simulink model "RPP_BankedDeePC"  (R2024a)
settings: Solver=FixedStepAuto  StartTime=0.0  StopTime=130  FixedStep=0.05  RelTol=1e-3
PostLoadFcn:
  | on_model_load
InitFcn:
  | on_model_start
StopFcn:
  | on_simulation_done
model workspace (MAT data in the model file):
  ActiveExperiment.Id = '1e727098-795b-40af-9168-30502f01196e'
  ActiveExperiment.Name = "Two steps"
  ActiveExperiment.Description = ""
  ActiveExperiment.ConstHorizonReference = 0
  ActiveExperiment.ComponentType = "scenario"
  ActiveExperiment.SimulationTime = 60
  ActiveExperiment.Subcomponents = "Disturbance"
  ActiveExperiment.Disturbance = struct()
  ActiveExperiment.SystemIc = [0; 0; 0; 0; 0; 0; 0; 0; 0; 0; 0; 0]
  ActiveExperiment.SystemParameterOverrides.payload_mass.timeseries__ = 1
  ActiveExperiment.SystemParameterOverrides.payload_mass.data = [0  0; 27  0]
  ActiveExperiment.Reference = '/home/luka/fer/csbenchlab_gym/envs/marine_otter_full/data/references/1e727098-795b-40af-9168-30502f01196e_ref.mat'
  ActiveExperiment.DisturbanceParameterOverrides = struct()
  ActiveExperiment.NumEvaluations = 1
  ActiveExperiment.RandomSeed = 42
  ActiveExperiment.SystemParams.payload_mass = timeseries
  ActiveExperiment.SystemParams.payload_mass.Name = 'unnamed'
  ActiveExperiment.SystemParams.payload_mass.DataInfo = tsdata.datametadata
  ActiveExperiment.SystemParams.payload_mass.DataInfo.Interpolation = tsdata.interpolation
  ActiveExperiment.SystemParams.payload_mass.DataInfo.Interpolation.Fhandle : function handle (value not decoded)
  ActiveExperiment.SystemParams.payload_mass.DataInfo.Interpolation.Name = 'linear'
  ActiveExperiment.SystemParams.payload_mass.TimeInfo = tsdata.timemetadata
  ActiveExperiment.SystemParams.payload_mass.TimeInfo.Length = 2
  ActiveExperiment.SystemParams.payload_mass.TimeInfo.DuplicateTimes = 0
  ActiveExperiment.SystemParams.payload_mass.TimeInfo.Time_ = [0; 27]
  ActiveExperiment.SystemParams.payload_mass.TimeInfo.Initialized = 1
  ActiveExperiment.SystemParams.payload_mass.QualityInfo = tsdata.qualmetadata
  ActiveExperiment.SystemParams.payload_mass.Data_ = [0; 0]
  ActiveExperiment.SystemParams.payload_location = timeseries
  ActiveExperiment.SystemParams.payload_location.Name = 'unnamed'
  ActiveExperiment.SystemParams.payload_location.DataInfo = tsdata.datametadata
  ActiveExperiment.SystemParams.payload_location.DataInfo.Interpolation = tsdata.interpolation
  ActiveExperiment.SystemParams.payload_location.DataInfo.Interpolation.Fhandle : function handle (value not decoded)
  ActiveExperiment.SystemParams.payload_location.DataInfo.Interpolation.Name = 'linear'
  ActiveExperiment.SystemParams.payload_location.TimeInfo = tsdata.timemetadata
  ActiveExperiment.SystemParams.payload_location.TimeInfo.Length = 1
  ActiveExperiment.SystemParams.payload_location.TimeInfo.DuplicateTimes = 0
  ActiveExperiment.SystemParams.payload_location.TimeInfo.Time_ = 0
  ActiveExperiment.SystemParams.payload_location.TimeInfo.Initialized = 1
  ActiveExperiment.SystemParams.payload_location.QualityInfo = tsdata.qualmetadata
  ActiveExperiment.SystemParams.payload_location.Data_ = [0; 0; 0]
  ActiveExperiment.SystemParams.current_speed = timeseries
  ActiveExperiment.SystemParams.current_speed.Name = 'unnamed'
  ActiveExperiment.SystemParams.current_speed.DataInfo = tsdata.datametadata
  ActiveExperiment.SystemParams.current_speed.DataInfo.Interpolation = tsdata.interpolation
  ActiveExperiment.SystemParams.current_speed.DataInfo.Interpolation.Fhandle : function handle (value not decoded)
  ActiveExperiment.SystemParams.current_speed.DataInfo.Interpolation.Name = 'linear'
  ActiveExperiment.SystemParams.current_speed.TimeInfo = tsdata.timemetadata
  ActiveExperiment.SystemParams.current_speed.TimeInfo.Length = 1
  ActiveExperiment.SystemParams.current_speed.TimeInfo.DuplicateTimes = 0
  ActiveExperiment.SystemParams.current_speed.TimeInfo.Time_ = 0
  ActiveExperiment.SystemParams.current_speed.TimeInfo.Initialized = 1
  ActiveExperiment.SystemParams.current_speed.QualityInfo = tsdata.qualmetadata
  ActiveExperiment.SystemParams.current_speed.Data_ = 0
  ActiveExperiment.SystemParams.current_direction = timeseries
  ActiveExperiment.SystemParams.current_direction.Name = 'unnamed'
  ActiveExperiment.SystemParams.current_direction.DataInfo = tsdata.datametadata
  ActiveExperiment.SystemParams.current_direction.DataInfo.Interpolation = tsdata.interpolation
  ActiveExperiment.SystemParams.current_direction.DataInfo.Interpolation.Fhandle : function handle (value not decoded)
  ActiveExperiment.SystemParams.current_direction.DataInfo.Interpolation.Name = 'linear'
  ActiveExperiment.SystemParams.current_direction.TimeInfo = tsdata.timemetadata
  ActiveExperiment.SystemParams.current_direction.TimeInfo.Length = 1
  ActiveExperiment.SystemParams.current_direction.TimeInfo.DuplicateTimes = 0
  ActiveExperiment.SystemParams.current_direction.TimeInfo.Time_ = 0
  ActiveExperiment.SystemParams.current_direction.TimeInfo.Initialized = 1
  ActiveExperiment.SystemParams.current_direction.QualityInfo = tsdata.qualmetadata
  ActiveExperiment.SystemParams.current_direction.Data_ = 0
  ActiveExperiment.SystemParams.out_gain = timeseries
  ActiveExperiment.SystemParams.out_gain.Name = 'unnamed'
  ActiveExperiment.SystemParams.out_gain.DataInfo = tsdata.datametadata
  ActiveExperiment.SystemParams.out_gain.DataInfo.Interpolation = tsdata.interpolation
  ActiveExperiment.SystemParams.out_gain.DataInfo.Interpolation.Fhandle : function handle (value not decoded)
  ActiveExperiment.SystemParams.out_gain.DataInfo.Interpolation.Name = 'linear'
  ActiveExperiment.SystemParams.out_gain.TimeInfo = tsdata.timemetadata
  ActiveExperiment.SystemParams.out_gain.TimeInfo.Length = 1
  ActiveExperiment.SystemParams.out_gain.TimeInfo.DuplicateTimes = 0
  ActiveExperiment.SystemParams.out_gain.TimeInfo.Time_ = 0
  ActiveExperiment.SystemParams.out_gain.TimeInfo.Initialized = 1
  ActiveExperiment.SystemParams.out_gain.QualityInfo = tsdata.qualmetadata
  ActiveExperiment.SystemParams.out_gain.Data_ = 1
  Experiments(1).Id = '1e1e735a-ca72-47f3-9e23-ef054322de06'
  Experiments(1).Name = "Five steps perturbed high noise"
  Experiments(1).Description = ""
  Experiments(1).ConstHorizonReference = 0
  Experiments(1).ComponentType = "scenario"
  Experiments(1).SimulationTime = 60
  Experiments(1).Subcomponents = "Disturbance"
  Experiments(1).Disturbance.Id = 'd00b25fa-299c-4dde-a026-233da86bc131'
  Experiments(1).Disturbance.Name = ''
  Experiments(1).Disturbance.Description = ''
  Experiments(1).Disturbance.LibVersionHash = ''
  Experiments(1).Disturbance.Lib = 'csbenchlab'
  Experiments(1).Disturbance.LibVersion = '0.0.1'
  Experiments(1).Disturbance.PluginType = 'dist'
  Experiments(1).Disturbance.PluginName = 'Gauss'
  Experiments(1).Disturbance.PluginImplementation = 'mat'
  Experiments(1).Disturbance.ParentComponentId = '1e1e735a-ca72-47f3-9e23-ef054322de06'
  Experiments(1).Disturbance.ParentComponentName = 'Five steps perturbed high noise'
  Experiments(1).Disturbance.ParentComponentType = 'scenario'
  Experiments(1).Disturbance.ComponentType = 'disturbance'
  Experiments(1).Disturbance.DestinationPath = 'disturbances'
  Experiments(1).SystemIc = [0; 0; 0; 0; 0; 0; 0; 0; 0; 0; 0; 0]
  Experiments(1).SystemParameterOverrides.payload_mass.timeseries__ = 1
  Experiments(1).SystemParameterOverrides.payload_mass.data = [0  35; 27  35]
  Experiments(1).Reference = '/home/luka/fer/csbenchlab_gym/envs/marine_otter_full/data/references/1e1e735a-ca72-47f3-9e23-ef054322de06_ref.mat'
  Experiments(1).DisturbanceParameterOverrides = struct()
  Experiments(1).NumEvaluations = 1000
  Experiments(1).RandomSeed = 42
  Experiments(2).Id = '1e727098-795b-40af-9168-30502f01196e'
  Experiments(2).Name = "Two steps"
  Experiments(2).Description = ""
  Experiments(2).ConstHorizonReference = 0
  Experiments(2).ComponentType = "scenario"
  Experiments(2).SimulationTime = 60
  Experiments(2).Subcomponents = "Disturbance"
  Experiments(2).Disturbance = struct()
  Experiments(2).SystemIc = [0; 0; 0; 0; 0; 0; 0; 0; 0; 0; 0; 0]
  Experiments(2).SystemParameterOverrides.payload_mass.timeseries__ = 1
  Experiments(2).SystemParameterOverrides.payload_mass.data = [0  0; 27  0]
  Experiments(2).Reference = '/home/luka/fer/csbenchlab_gym/envs/marine_otter_full/data/references/1e727098-795b-40af-9168-30502f01196e_ref.mat'
  Experiments(2).DisturbanceParameterOverrides = struct()
  Experiments(2).NumEvaluations = 1
  Experiments(2).RandomSeed = 42
  Experiments(3).Id = '832a0fb6-0823-4b09-93b7-a1f8c841e784'
  Experiments(3).Name = "Sinuses"
  Experiments(3).Description = ""
  Experiments(3).ConstHorizonReference = 0
  Experiments(3).ComponentType = "scenario"
  Experiments(3).SimulationTime = 60
  Experiments(3).Subcomponents = "Disturbance"
  Experiments(3).Disturbance.Id = '6582568e-6a07-4ca1-973d-ce726013b9e5'
  Experiments(3).Disturbance.Name = ''
  Experiments(3).Disturbance.Description = ''
  Experiments(3).Disturbance.LibVersionHash = ''
  Experiments(3).Disturbance.Lib = 'csbenchlab'
  Experiments(3).Disturbance.LibVersion = '0.0.1'
  Experiments(3).Disturbance.PluginType = 'dist'
  Experiments(3).Disturbance.PluginName = 'Gauss'
  Experiments(3).Disturbance.PluginImplementation = 'mat'
  Experiments(3).Disturbance.ParentComponentId = '832a0fb6-0823-4b09-93b7-a1f8c841e784'
  Experiments(3).Disturbance.ParentComponentName = 'Sinuses'
  Experiments(3).Disturbance.ParentComponentType = 'scenario'
  Experiments(3).Disturbance.ComponentType = 'disturbance'
  Experiments(3).Disturbance.DestinationPath = 'disturbances'
  Experiments(3).SystemIc = [0; 0; 0; 0; 0; 0; 0; 0; 0; 0; 0; 0]
  Experiments(3).SystemParameterOverrides.payload_mass.timeseries__ = 1
  Experiments(3).SystemParameterOverrides.payload_mass.data = [0  35; 12  35]
  Experiments(3).Reference = '/home/luka/fer/csbenchlab_gym/envs/marine_otter_full/data/references/832a0fb6-0823-4b09-93b7-a1f8c841e784_ref.mat'
  Experiments(3).DisturbanceParameterOverrides = struct()
  Experiments(3).NumEvaluations = 1000
  Experiments(3).RandomSeed = 42
  Experiments(4).Id = '85ae8ae8-3421-447e-86e6-f1860a57dbe5'
  Experiments(4).Name = "Two steps high noise"
  Experiments(4).Description = ""
  Experiments(4).ConstHorizonReference = 0
  Experiments(4).ComponentType = "scenario"
  Experiments(4).SimulationTime = 60
  Experiments(4).Subcomponents = "Disturbance"
  Experiments(4).Disturbance.Id = 'ccaeaedb-34fb-4469-93e3-0e771cb356d7'
  Experiments(4).Disturbance.Name = 'New Disturbance'
  Experiments(4).Disturbance.Description = ''
  Experiments(4).Disturbance.LibVersionHash = ''
  Experiments(4).Disturbance.Lib = 'csbenchlab'
  Experiments(4).Disturbance.LibVersion = '0.0.1'
  Experiments(4).Disturbance.PluginType = 'dist'
  Experiments(4).Disturbance.PluginName = 'Gauss'
  Experiments(4).Disturbance.PluginImplementation = 'mat'
  Experiments(4).Disturbance.ParentComponentId = '85ae8ae8-3421-447e-86e6-f1860a57dbe5'
  Experiments(4).Disturbance.ParentComponentType = 'scenario'
  Experiments(4).Disturbance.ComponentType = 'disturbance'
  Experiments(4).Disturbance.ParentComponentName = 'Two steps high noise'
  Experiments(4).SystemIc = [0; 0; 0; 0; 0; 0; 0; 0; 0; 0; 0; 0]
  Experiments(4).SystemParameterOverrides.payload_mass.timeseries__ = 1
  Experiments(4).SystemParameterOverrides.payload_mass.data = [0  0; 30  20]
  Experiments(4).SystemParameterOverrides.payload_location.timeseries__ = 1
  Experiments(4).SystemParameterOverrides.payload_location.data = [0 0 -0.15 0]
  Experiments(4).SystemParameterOverrides.current_speed = 0.2
  Experiments(4).SystemParameterOverrides.current_direction = 0.1
  Experiments(4).Reference = '/home/luka/fer/csbenchlab_gym/envs/marine_otter_full/data/references/85ae8ae8-3421-447e-86e6-f1860a57dbe5_ref.mat'
  Experiments(4).DisturbanceParameterOverrides = struct()
  Experiments(4).NumEvaluations = 1
  Experiments(4).RandomSeed = 42
  Experiments(5).Id = '9caafca7-6b3d-4fd5-b43b-2d0badebda60'
  Experiments(5).Name = "Five steps perturbed"
  Experiments(5).Description = ""
  Experiments(5).ConstHorizonReference = 0
  Experiments(5).ComponentType = "scenario"
  Experiments(5).SimulationTime = 60
  Experiments(5).Subcomponents = "Disturbance"
  Experiments(5).Disturbance.Id = '941af73e-12e7-42cf-853d-f79bb40068e7'
  Experiments(5).Disturbance.Name = ''
  Experiments(5).Disturbance.Description = ''
  Experiments(5).Disturbance.LibVersionHash = ''
  Experiments(5).Disturbance.Lib = 'csbenchlab'
  Experiments(5).Disturbance.LibVersion = '0.0.1'
  Experiments(5).Disturbance.PluginType = 'dist'
  Experiments(5).Disturbance.PluginName = 'Gauss'
  Experiments(5).Disturbance.PluginImplementation = 'mat'
  Experiments(5).Disturbance.ParentComponentId = '9caafca7-6b3d-4fd5-b43b-2d0badebda60'
  Experiments(5).Disturbance.ParentComponentName = 'Five steps perturbed'
  Experiments(5).Disturbance.ParentComponentType = 'scenario'
  Experiments(5).Disturbance.ComponentType = 'disturbance'
  Experiments(5).Disturbance.DestinationPath = 'disturbances'
  Experiments(5).SystemIc = [0; 0; 0; 0; 0; 0; 0; 0; 0; 0; 0; 0]
  Experiments(5).SystemParameterOverrides.payload_mass.timeseries__ = 1
  Experiments(5).SystemParameterOverrides.payload_mass.data = [0  0; 27  0]
  Experiments(5).Reference = '/home/luka/fer/csbenchlab_gym/envs/marine_otter_full/data/references/9caafca7-6b3d-4fd5-b43b-2d0badebda60_ref.mat'
  Experiments(5).DisturbanceParameterOverrides = struct()
  Experiments(5).NumEvaluations = 1000
  Experiments(5).RandomSeed = 42
  Experiments(6).Id = 'd997722b-b22e-4a88-a68f-d421073cfd81'
  Experiments(6).Name = "Sinuses high noise"
  Experiments(6).Description = ""
  Experiments(6).ConstHorizonReference = 0
  Experiments(6).ComponentType = "scenario"
  Experiments(6).SimulationTime = 60
  Experiments(6).Subcomponents = "Disturbance"
  Experiments(6).Disturbance.Id = 'e3fab669-38a8-480e-9185-300544970487'
  Experiments(6).Disturbance.Name = ''
  Experiments(6).Disturbance.Description = ''
  Experiments(6).Disturbance.LibVersionHash = ''
  Experiments(6).Disturbance.Lib = 'csbenchlab'
  Experiments(6).Disturbance.LibVersion = '0.0.1'
  Experiments(6).Disturbance.PluginType = 'dist'
  Experiments(6).Disturbance.PluginName = 'Gauss'
  Experiments(6).Disturbance.PluginImplementation = 'mat'
  Experiments(6).Disturbance.ParentComponentId = 'd997722b-b22e-4a88-a68f-d421073cfd81'
  Experiments(6).Disturbance.ParentComponentName = 'Sinuses high noise'
  Experiments(6).Disturbance.ParentComponentType = 'scenario'
  Experiments(6).Disturbance.ComponentType = 'disturbance'
  Experiments(6).Disturbance.DestinationPath = 'disturbances'
  Experiments(6).SystemIc = [0; 0; 0; 0; 0; 0; 0; 0; 0; 0; 0; 0]
  Experiments(6).SystemParameterOverrides.payload_mass.timeseries__ = 1
  Experiments(6).SystemParameterOverrides.payload_mass.data = [0  35; 12  35]
  Experiments(6).Reference = '/home/luka/fer/csbenchlab_gym/envs/marine_otter_full/data/references/d997722b-b22e-4a88-a68f-d421073cfd81_ref.mat'
  Experiments(6).DisturbanceParameterOverrides = struct()
  Experiments(6).NumEvaluations = 1000
  Experiments(6).RandomSeed = 42
  GlobalReference = 0
  RPP_BankedDeePC_CS_Controller_BankedDeePC_d_data.Ts = 0.05
  RPP_BankedDeePC_CS_Controller_BankedDeePC_d_data.T = 100
  RPP_BankedDeePC_CS_Controller_BankedDeePC_d_data.m = 2
  RPP_BankedDeePC_CS_Controller_BankedDeePC_d_data.p = 2
  RPP_BankedDeePC_CS_Controller_BankedDeePC_d_data.L = 12
  RPP_BankedDeePC_CS_Controller_BankedDeePC_d_data.Tini = 5
  RPP_BankedDeePC_CS_Controller_BankedDeePC_d_data.vel_stop_idx = 2
  RPP_BankedDeePC_CS_Controller_BankedDeePC_d_data.idx.m = 2
  RPP_BankedDeePC_CS_Controller_BankedDeePC_d_data.idx.p = 2
  RPP_BankedDeePC_CS_Controller_BankedDeePC_d_data.idx.L = 12
  RPP_BankedDeePC_CS_Controller_BankedDeePC_d_data.idx.Tini = 5
  RPP_BankedDeePC_CS_Controller_BankedDeePC_d_data.idx.uini_v.b = 1
  RPP_BankedDeePC_CS_Controller_BankedDeePC_d_data.idx.uini_v.e = 10
  RPP_BankedDeePC_CS_Controller_BankedDeePC_d_data.idx.uini_v.sz = 10
  RPP_BankedDeePC_CS_Controller_BankedDeePC_d_data.idx.uini_v.r = [1 2 3 4 5 6 7 8 9 10]
  RPP_BankedDeePC_CS_Controller_BankedDeePC_d_data.idx.u_v.b = 11
  RPP_BankedDeePC_CS_Controller_BankedDeePC_d_data.idx.u_v.e = 34
  RPP_BankedDeePC_CS_Controller_BankedDeePC_d_data.idx.u_v.sz = 24
  RPP_BankedDeePC_CS_Controller_BankedDeePC_d_data.idx.u_v.r = [11 12 13 14 15 16 17 18 19 20 21 22 23 24 25 26 27 28 29 30 31 32 33 34]
  RPP_BankedDeePC_CS_Controller_BankedDeePC_d_data.idx.yini_v.b = 35
  RPP_BankedDeePC_CS_Controller_BankedDeePC_d_data.idx.yini_v.e = 44
  RPP_BankedDeePC_CS_Controller_BankedDeePC_d_data.idx.yini_v.sz = 10
  RPP_BankedDeePC_CS_Controller_BankedDeePC_d_data.idx.yini_v.r = [35 36 37 38 39 40 41 42 43 44]
  RPP_BankedDeePC_CS_Controller_BankedDeePC_d_data.idx.y_v.b = 45
  RPP_BankedDeePC_CS_Controller_BankedDeePC_d_data.idx.y_v.e = 68
  RPP_BankedDeePC_CS_Controller_BankedDeePC_d_data.idx.y_v.sz = 24
  RPP_BankedDeePC_CS_Controller_BankedDeePC_d_data.idx.y_v.r = [45 46 47 48 49 50 51 52 53 54 55 56 57 58 59 60 61 62 63 64 65 66 67 68]
  RPP_BankedDeePC_CS_Controller_BankedDeePC_d_data.idx.u.b = 1
  RPP_BankedDeePC_CS_Controller_BankedDeePC_d_data.idx.u.e = 24
  RPP_BankedDeePC_CS_Controller_BankedDeePC_d_data.idx.u.sz = 24
  RPP_BankedDeePC_CS_Controller_BankedDeePC_d_data.idx.u.r = [1 2 3 4 5 6 7 8 9 10 11 12 13 14 15 16 17 18 19 20 21 22 23 24]
  RPP_BankedDeePC_CS_Controller_BankedDeePC_d_data.idx.y.b = 25
  RPP_BankedDeePC_CS_Controller_BankedDeePC_d_data.idx.y.e = 48
  RPP_BankedDeePC_CS_Controller_BankedDeePC_d_data.idx.y.sz = 24
  RPP_BankedDeePC_CS_Controller_BankedDeePC_d_data.idx.y.r = [25 26 27 28 29 30 31 32 33 34 35 36 37 38 39 40 41 42 43 44 45 46 47 48]
  RPP_BankedDeePC_CS_Controller_BankedDeePC_d_data.idx.s.b = 49
  RPP_BankedDeePC_CS_Controller_BankedDeePC_d_data.idx.s.e = 82
  RPP_BankedDeePC_CS_Controller_BankedDeePC_d_data.idx.s.sz = 34
  RPP_BankedDeePC_CS_Controller_BankedDeePC_d_data.idx.s.r = [49 50 51 52 53 54 55 56 57 58 59 60 61 62 63 64 65 66 67 68 69 70 71 72 73 74 75 76 77 78 79 80 81 82]
  RPP_BankedDeePC_CS_Controller_BankedDeePC_d_data.idx.A_v.b = 1
  RPP_BankedDeePC_CS_Controller_BankedDeePC_d_data.idx.A_v.e = 68
  RPP_BankedDeePC_CS_Controller_BankedDeePC_d_data.idx.A_v.sz = 68
  RPP_BankedDeePC_CS_Controller_BankedDeePC_d_data.idx.A_v.r = [1 2 3 4 5 6 7 8 9 10 11 12 13 14 15 16 17 18 19 20 21 22 23 24 25 26 27 28 29 30 31 32 33 34 35 36 37 38 39 40 41 42 43 44 45 46 47 48 49 50 51 52 53 54 55 56 57 58 59 60 61 62 63 64 65 66 67 68]
  RPP_BankedDeePC_CS_Controller_BankedDeePC_d_data.idx.yterm.b = 83
  RPP_BankedDeePC_CS_Controller_BankedDeePC_d_data.idx.yterm.e = 84
  RPP_BankedDeePC_CS_Controller_BankedDeePC_d_data.idx.yterm.sz = 2
  RPP_BankedDeePC_CS_Controller_BankedDeePC_d_data.idx.yterm.r = [83 84]
  RPP_BankedDeePC_CS_Controller_BankedDeePC_d_data.idx.uterm.b = 85
  RPP_BankedDeePC_CS_Controller_BankedDeePC_d_data.idx.uterm.e = 86
  RPP_BankedDeePC_CS_Controller_BankedDeePC_d_data.idx.uterm.sz = 2
  RPP_BankedDeePC_CS_Controller_BankedDeePC_d_data.idx.uterm.r = [85 86]
  RPP_BankedDeePC_CS_Controller_BankedDeePC_d_data.idx.uterm_v.b = 72
  RPP_BankedDeePC_CS_Controller_BankedDeePC_d_data.idx.uterm_v.e = 73
  RPP_BankedDeePC_CS_Controller_BankedDeePC_d_data.idx.uterm_v.sz = 2
  RPP_BankedDeePC_CS_Controller_BankedDeePC_d_data.idx.uterm_v.r = [72 73]
  RPP_BankedDeePC_CS_Controller_BankedDeePC_d_data.idx.yterm_v.b = 70
  RPP_BankedDeePC_CS_Controller_BankedDeePC_d_data.idx.yterm_v.e = 71
  RPP_BankedDeePC_CS_Controller_BankedDeePC_d_data.idx.yterm_v.sz = 2
  RPP_BankedDeePC_CS_Controller_BankedDeePC_d_data.idx.yterm_v.r = [70 71]
  RPP_BankedDeePC_CS_Controller_BankedDeePC_d_data.idx.affine_v.b = 69
  RPP_BankedDeePC_CS_Controller_BankedDeePC_d_data.idx.affine_v.e = 69
  RPP_BankedDeePC_CS_Controller_BankedDeePC_d_data.idx.affine_v.sz = 1
  RPP_BankedDeePC_CS_Controller_BankedDeePC_d_data.idx.affine_v.r = 69
  RPP_BankedDeePC_CS_Controller_BankedDeePC_d_data.idx.total_constraints = 5
  RPP_BankedDeePC_CS_Controller_BankedDeePC_d_data.idx.term_v.b = 69
  RPP_BankedDeePC_CS_Controller_BankedDeePC_d_data.idx.term_v.e = 73
  RPP_BankedDeePC_CS_Controller_BankedDeePC_d_data.idx.term_v.sz = 5
  RPP_BankedDeePC_CS_Controller_BankedDeePC_d_data.idx.term_v.r = [69 70 71 72 73]
  RPP_BankedDeePC_CS_Controller_BankedDeePC_d_data.idx.a.b = 87
  RPP_BankedDeePC_CS_Controller_BankedDeePC_d_data.idx.a.e = 170
  RPP_BankedDeePC_CS_Controller_BankedDeePC_d_data.idx.a.sz = 84
  RPP_BankedDeePC_CS_Controller_BankedDeePC_d_data.idx.a.r = [87 88 89 90 91 92 93 94 95 96 97 98 99 100 101 102 103 104 105 106 107 108 109 110 111 112 113 114 115 116 117 118 119 120 121 122 123 124 125 126 127 128 129 130 131 132 133 134 135 136 137 138 139 140 141 142 143 144 145 146 147 148 149 150 151 152 153 154 155 156 157 158 159 160 161 162 163 164 165 166 167 168 169 170]
  RPP_BankedDeePC_CS_Controller_BankedDeePC_d_data.idx.state.b = 1
  RPP_BankedDeePC_CS_Controller_BankedDeePC_d_data.idx.state.e = 170
  RPP_BankedDeePC_CS_Controller_BankedDeePC_d_data.idx.state.sz = 170
  RPP_BankedDeePC_CS_Controller_BankedDeePC_d_data.idx.state.r = [1 2 3 4 5 6 7 8 9 10 11 12 13 14 15 16 17 18 19 20 21 22 23 24 25 26 27 28 29 30 31 32 33 34 35 36 37 38 39 40 41 42 43 44 45 46 47 48 49 50 51 52 53 54 55 56 57 58 59 60 61 62 63 64 65 66 67 68 69 70 71 72 73 74 75 76 77 78 79 80 81 82 83 84 85 86 87 88 89 90 91 92 93 94 95 96 97 98 99 100 101 102 103 104 105 106 107 108 109 110 111 112 113 114 115 116 117 118 119 120 121 122 123 124 125 126 127 128 129 130 131 132 133 134 135 136 137 138 139 140 141 142 143 144 145 146 147 148 149 150 151 152 153 154 155 156 157 158 159 160 161 162 163 164 165 166 167 168 169 170]
  RPP_BankedDeePC_CS_Controller_BankedDeePC_d_data.idx.u_lt.b = 1
  RPP_BankedDeePC_CS_Controller_BankedDeePC_d_data.idx.u_lt.e = 48
  RPP_BankedDeePC_CS_Controller_BankedDeePC_d_data.idx.u_lt.sz = 48
  RPP_BankedDeePC_CS_Controller_BankedDeePC_d_data.idx.u_lt.r = [1 2 3 4 5 6 7 8 9 10 11 12 13 14 15 16 17 18 19 20 21 22 23 24 25 26 27 28 29 30 31 32 33 34 35 36 37 38 39 40 41 42 43 44 45 46 47 48]
  RPP_BankedDeePC_CS_Controller_BankedDeePC_d_data.idx.y_lt.b = -1
  RPP_BankedDeePC_CS_Controller_BankedDeePC_d_data.idx.y_lt.e = -1
  RPP_BankedDeePC_CS_Controller_BankedDeePC_d_data.idx.y_lt.sz = 1
  RPP_BankedDeePC_CS_Controller_BankedDeePC_d_data.idx.y_lt.r = -1
  RPP_BankedDeePC_CS_Controller_BankedDeePC_d_data.x_op_u = [0; 0; 0; 0; 0; 0; 0; 0; 0; 0; 0; 0; 0; 0; 0; 0; 0; 0; 0; 0; 0; 0; 0; 0]
  RPP_BankedDeePC_CS_Controller_BankedDeePC_d_data.x_op_y = [0; 0; 0; 0; 0; 0; 0; 0; 0; 0; 0; 0; 0; 0; 0; 0; 0; 0; 0; 0; 0; 0; 0; 0]
  RPP_BankedDeePC_CS_Controller_BankedDeePC_d_data.x_op_g = [0; 0; 0; 0; 0; 0; 0; 0; 0; 0; 0; 0; 0; 0; 0; 0; 0; 0; 0; 0; 0; 0; 0; 0; 0; 0; 0; 0; 0; 0; 0; 0; 0; 0; 0; 0; 0; 0; 0; 0; 0; 0; 0; 0; 0; 0; 0; 0; 0; 0; 0; 0; 0; 0; 0; 0; 0; 0; 0; 0; 0; 0; 0; 0; 0; 0; 0; 0; 0; 0; 0; 0; 0; 0; 0; 0; 0; 0; 0; 0; 0; 0; 0; 0]
  RPP_BankedDeePC_CS_Controller_BankedDeePC_d_data.uini = [0; 0; 0; 0; 0; 0; 0; 0; 0; 0]
  RPP_BankedDeePC_CS_Controller_BankedDeePC_d_data.yini = [0; 0; 0; 0; 0; 0; 0; 0; 0; 0]
  RPP_BankedDeePC_CS_Controller_BankedDeePC_d_data.A = [0 0 0 0 0 0 0 0 0 0 -1 0 ... (12410 elements, 73x170)]
  RPP_BankedDeePC_CS_Controller_BankedDeePC_d_data.b = [0; 0; 0; 0; 0; 0; 0; 0; 0; 0; 0; 0; 0; 0; 0; 0; 0; 0; 0; 0; 0; 0; 0; 0; 0; 0; 0; 0; 0; 0; 0; 0; 0; 0; 0; 0; 0; 0; 0; 0; 0; 0; 0; 0; 0; 0; 0; 0; 0; 0; 0; 0; 0; 0; 0; 0; 0; 0; 0; 0; 0; 0; 0; 0; 0; 0; 0; 0; 1; 0; 0; 0; 0]
  RPP_BankedDeePC_CS_Controller_BankedDeePC_d_data.A_lt = [1 0 -1 0 -1 0 1 0 0 0 0 0 ... (8160 elements, 48x170)]
  RPP_BankedDeePC_CS_Controller_BankedDeePC_d_data.b_lt = [0.2; 0.2; 0.2; 0.2; 0.2; 0.2; 0.2; 0.2; 0.2; 0.2; 0.2; 0.2; 0.2; 0.2; 0.2; 0.2; 0.2; 0.2; 0.2; 0.2; 0.2; 0.2; 0.2; 0.2; 0.2; 0.2; 0.2; 0.2; 0.2; 0.2; 0.2; 0.2; 0.2; 0.2; 0.2; 0.2; 0.2; 0.2; 0.2; 0.2; 0.2; 0.2; 0.2; 0.2; 0.2; 0.2; 0.2; 0.2]
  RPP_BankedDeePC_CS_Controller_BankedDeePC_d_data.optim_T = [0.0666666666667 0 0 0 0 0 0 0 0 0 0 0 ... (28900 elements, 170x170)]
  RPP_BankedDeePC_CS_Controller_BankedDeePC_d_data.optim_f = [0; 0; 0; 0; 0; 0; 0; 0; 0; 0; 0; 0; 0; 0; 0; 0; 0; 0; 0; 0; 0; 0; 0; 0; 0; 0; 0; 0; 0; 0; 0; 0; 0; 0; 0; 0; 0; 0; 0; 0; 0; 0; 0; 0; 0; 0; 0; 0; 0; 0; 0; 0; 0; 0; 0; 0; 0; 0; 0; 0; 0; 0; 0; 0; 0; 0; 0; 0; 0; 0; 0; 0; 0; 0; 0; 0; 0; 0; 0; 0; 0; 0; 0; 0; 0; 0; 0; 0; 0; 0; 0; 0; 0; 0; 0; 0; 0; 0; 0; 0; 0; 0; 0; 0; 0; 0; 0; 0; 0; 0; 0; 0; 0; 0; 0; 0; 0; 0; 0; 0; 0; 0; 0; 0; 0; 0; 0; 0; 0; 0; 0; 0; 0; 0; 0; 0; 0; 0; 0; 0; 0; 0; 0; 0; 0; 0; 0; 0; 0; 0; 0; 0; 0; 0; 0; 0; 0; 0; 0; 0; 0; 0; 0; 0; 0; 0; 0; 0; 0; 0]
  RPP_BankedDeePC_CS_Controller_BankedDeePC_d_data.x_op = [0; 0; 0; 0; 0; 0; 0; 0; 0; 0; 0; 0; 0; 0; 0; 0; 0; 0; 0; 0; 0; 0; 0; 0; 0; 0; 0; 0; 0; 0; 0; 0; 0; 0; 0; 0; 0; 0; 0; 0; 0; 0; 0; 0; 0; 0; 0; 0; 0; 0; 0; 0; 0; 0; 0; 0; 0; 0; 0; 0; 0; 0; 0; 0; 0; 0; 0; 0; 0; 0; 0; 0; 0; 0; 0; 0; 0; 0; 0; 0; 0; 0; 0; 0; 0; 0; 0; 0; 0; 0; 0; 0; 0; 0; 0; 0; 0; 0; 0; 0; 0; 0; 0; 0; 0; 0; 0; 0; 0; 0; 0; 0; 0; 0; 0; 0; 0; 0; 0; 0; 0; 0; 0; 0; 0; 0; 0; 0; 0; 0; 0; 0; 0; 0; 0; 0; 0; 0; 0; 0; 0; 0; 0; 0; 0; 0; 0; 0; 0; 0; 0; 0; 0; 0; 0; 0; 0; 0; 0; 0; 0; 0; 0; 0; 0; 0; 0; 0; 0; 0]
  RPP_BankedDeePC_CS_Controller_BankedDeePC_d_data.lb = [-Inf; -Inf; -Inf; -Inf; -Inf; -Inf; -Inf; -Inf; -Inf; -Inf; -Inf; -Inf; -Inf; -Inf; -Inf; -Inf; -Inf; -Inf; -Inf; -Inf; -Inf; -Inf; -Inf; -Inf; -Inf; -Inf; -Inf; -Inf; -Inf; -Inf; -Inf; -Inf; -Inf; -Inf; -Inf; -Inf; -Inf; -Inf; -Inf; -Inf; -Inf; -Inf; -Inf; -Inf; -Inf; -Inf; -Inf; -Inf; -Inf; -Inf; -Inf; -Inf; -Inf; -Inf; -Inf; -Inf; -Inf; -Inf; -Inf; -Inf; -Inf; -Inf; -Inf; -Inf; -Inf; -Inf; -Inf; -Inf; -Inf; -Inf; -Inf; -Inf; -Inf; -Inf; -Inf; -Inf; -Inf; -Inf; -Inf; -Inf; -Inf; -Inf; -Inf; -Inf; -Inf; -Inf; -Inf; -Inf; -Inf; -Inf; -Inf; -Inf; -Inf; -Inf; -Inf; -Inf; -Inf; -Inf; -Inf; -Inf; -Inf; -Inf; -Inf; -Inf; -Inf; -Inf; -Inf; -Inf; -Inf; -Inf; -Inf; -Inf; -Inf; -Inf; -Inf; -Inf; -Inf; -Inf; -Inf; -Inf; -Inf; -Inf; -Inf; -Inf; -Inf; -Inf; -Inf; -Inf; -Inf; -Inf; -Inf; -Inf; -Inf; -Inf; -Inf; -Inf; -Inf; -Inf; -Inf; -Inf; -Inf; -Inf; -Inf; -Inf; -Inf; -Inf; -Inf; -Inf; -Inf; -Inf; -Inf; -Inf; -Inf; -Inf; -Inf; -Inf; -Inf; -Inf; -Inf; -Inf; -Inf; -Inf; -Inf; -Inf; -Inf; -Inf; -Inf; -Inf; -Inf; -Inf]
  RPP_BankedDeePC_CS_Controller_BankedDeePC_d_data.ub = [Inf; Inf; Inf; Inf; Inf; Inf; Inf; Inf; Inf; Inf; Inf; Inf; Inf; Inf; Inf; Inf; Inf; Inf; Inf; Inf; Inf; Inf; Inf; Inf; Inf; Inf; Inf; Inf; Inf; Inf; Inf; Inf; Inf; Inf; Inf; Inf; Inf; Inf; Inf; Inf; Inf; Inf; Inf; Inf; Inf; Inf; Inf; Inf; Inf; Inf; Inf; Inf; Inf; Inf; Inf; Inf; Inf; Inf; Inf; Inf; Inf; Inf; Inf; Inf; Inf; Inf; Inf; Inf; Inf; Inf; Inf; Inf; Inf; Inf; Inf; Inf; Inf; Inf; Inf; Inf; Inf; Inf; Inf; Inf; Inf; Inf; Inf; Inf; Inf; Inf; Inf; Inf; Inf; Inf; Inf; Inf; Inf; Inf; Inf; Inf; Inf; Inf; Inf; Inf; Inf; Inf; Inf; Inf; Inf; Inf; Inf; Inf; Inf; Inf; Inf; Inf; Inf; Inf; Inf; Inf; Inf; Inf; Inf; Inf; Inf; Inf; Inf; Inf; Inf; Inf; Inf; Inf; Inf; Inf; Inf; Inf; Inf; Inf; Inf; Inf; Inf; Inf; Inf; Inf; Inf; Inf; Inf; Inf; Inf; Inf; Inf; Inf; Inf; Inf; Inf; Inf; Inf; Inf; Inf; Inf; Inf; Inf; Inf; Inf; Inf; Inf; Inf; Inf; Inf; Inf]
  RPP_BankedDeePC_CS_Controller_BankedDeePC_d_data.fval = 0
  RPP_BankedDeePC_CS_Controller_BankedDeePC_d_data.old_y_ref = [0; 0]
  RPP_BankedDeePC_CS_Controller_BankedDeePC_d_data.eta = [0; 0]
  RPP_BankedDeePC_CS_Controller_BankedDeePC_d_data.has_lt = 1
  callbacks = dictionary
  callbacks.data.Version = 1
  callbacks.data.IsKeyCombined = 1
  callbacks.data.IsValueCombined = 1
  callbacks.data.Key = ["on_start:31b52d05-ccc9-4eab-bb0e-3c80b4e6f477"; "on_start:f41ef9e4-ba34-416c-84b6-7794956a3c04"; "on_start:9c40ba40-a30c-4d47-b6ea-332d53085db4"; "on_start:a6a9c6d3-ff58-4f5d-b7b7-6a5809d04cef"; "on_start:59d3b695-31bd-4d38-a8d0-9c2b61ca3ebd"; "on_start:68187f7d-81f5-4756-96be-de0d65363a63"; "on_start:17c1b7c7-d1b2-4e6c-bab6-21ffb9ee4dcb"; "on_start:a5c8738f-8d38-4797-a21a-203fc6d46076"; "on_load:4a0d1010-4549-4d51-b3a5-602e7c932b45"; "on_start:4a0d1010-4549-4d51-b3a5-602e7c932b45"; "on_end:4a0d1010-4549-4d51-b3a5-602e7c932b45"]
  callbacks.data.Value{1}.external_function__ = 1
  callbacks.data.Value{1}.function = 'configure_controller_params'
  callbacks.data.Value{1}.backend = 'm'
  callbacks.data.Value{1}.kwargs = struct()
  callbacks.data.Value{2}.external_function__ = 1
  callbacks.data.Value{2}.function = 'configure_controller_params'
  callbacks.data.Value{2}.backend = 'm'
  callbacks.data.Value{2}.kwargs = struct()
  callbacks.data.Value{3}.external_function__ = 1
  callbacks.data.Value{3}.function = 'configure_controller_params'
  callbacks.data.Value{3}.backend = 'm'
  callbacks.data.Value{3}.kwargs = struct()
  callbacks.data.Value{4}.external_function__ = 1
  callbacks.data.Value{4}.function = 'configure_controller_params'
  callbacks.data.Value{4}.backend = 'm'
  callbacks.data.Value{4}.kwargs = struct()
  callbacks.data.Value{5}.external_function__ = 1
  callbacks.data.Value{5}.function = 'configure_controller_params'
  callbacks.data.Value{5}.backend = 'm'
  callbacks.data.Value{5}.kwargs = struct()
  callbacks.data.Value{6}.external_function__ = 1
  callbacks.data.Value{6}.function = 'configure_controller_params'
  callbacks.data.Value{6}.backend = 'm'
  callbacks.data.Value{6}.kwargs = struct()
  callbacks.data.Value{7}.external_function__ = 1
  callbacks.data.Value{7}.function = 'configure_controller_params'
  callbacks.data.Value{7}.backend = 'm'
  callbacks.data.Value{7}.kwargs = struct()
  callbacks.data.Value{8}.external_function__ = 1
  callbacks.data.Value{8}.function = 'configure_controller_params'
  callbacks.data.Value{8}.backend = 'm'
  callbacks.data.Value{8}.kwargs = struct()
  callbacks.data.Value{9} = py.function
  callbacks.data.Value{10} = py.function
  callbacks.data.Value{11} = py.function
  env_name = 'RPP_BankedDeePC'
  extrinsic = 1
  gen_blocks : object (value not decoded)
  gen_data_dictionary = Simulink.data.Dictionary
  id_to_params_path_map = dictionary
  id_to_params_path_map.data.Version = 1
  id_to_params_path_map.data.IsKeyCombined = 1
  id_to_params_path_map.data.IsValueCombined = 1
  id_to_params_path_map.data.Key = ["4a0d1010-4549-4d51-b3a5-602e7c932b45"; "9c40ba40-a30c-4d47-b6ea-332d53085db4"; "d00b25fa-299c-4dde-a026-233da86bc131"; "6582568e-6a07-4ca1-973d-ce726013b9e5"; "ccaeaedb-34fb-4469-93e3-0e771cb356d7"; "941af73e-12e7-42cf-853d-f79bb40068e7"; "e3fab669-38a8-480e-9185-300544970487"]
  id_to_params_path_map.data.Value = ["RPP_BankedDeePC_params.sys.Otter"; "RPP_BankedDeePC_params.ctl.BankedDeePC_d"; "RPP_BankedDeePC_params.Subcomponents.FiveStepsPerturbedHighNoise.x"; "RPP_BankedDeePC_params.Subcomponents.Sinuses.x"; "RPP_BankedDeePC_params.Subcomponents.TwoStepsHighNoise.NewDisturbance"; "RPP_BankedDeePC_params.Subcomponents.FiveStepsPerturbed.x"; "RPP_BankedDeePC_params.Subcomponents.SinusesHighNoise.x"]
  model_info.Metadata.Id = "ab4d190f-a5ed-423c-bf24-5e5b13858970"
  model_info.Metadata.Name = "marine_otter_full"
  model_info.Metadata.Version = "0.1"
  model_info.Metadata.Ts = 0.05
  model_info.Metadata.ComponentType = "metadata"
  model_info.Metadata.CoderExtrinsic = 1
  model_info.Controllers.Id = "9c40ba40-a30c-4d47-b6ea-332d53085db4"
  model_info.Controllers.Name = "BankedDeePC_d"
  model_info.Controllers.Description = ""
  model_info.Controllers.LibVersionHash = ""
  model_info.Controllers.Lib = "data_driven_lib"
  model_info.Controllers.LibVersion = "0.0.1"
  model_info.Controllers.PluginType = "ctl"
  model_info.Controllers.PluginName = "BankedDeePC"
  model_info.Controllers.IsComposable = 0
  model_info.Controllers.RefHorizon = 10
  model_info.Controllers.Mux.Inputs = [1 6]
  model_info.Controllers.Mux.Outputs = [1 2]
  model_info.Controllers.Subcomponents = ["Disturbance" "Subcontrollers"]
  model_info.Controllers.Disturbance = struct()
  model_info.Controllers.ComponentType = "controller"
  model_info.Controllers.PluginImplementation = "mat"
  model_info.Controllers.Subcontrollers = struct()
  model_info.System.Id = "4a0d1010-4549-4d51-b3a5-602e7c932b45"
  model_info.System.Name = "Otter"
  model_info.System.Description = ""
  model_info.System.LibVersionHash = ""
  model_info.System.Lib = "marine_lib"
  model_info.System.LibVersion = "0.0.1"
  model_info.System.PluginType = "sys"
  model_info.System.PluginName = "Otter"
  model_info.System.Subcomponents = "Disturbance"
  model_info.System.Disturbance = struct()
  model_info.System.ComponentType = "system"
  model_info.System.PluginImplementation = "slx"
  model_info.Metrics.Id = "9c8fc09b-5b47-4f25-8326-e915b50c92f8"
  model_info.Metrics.Name = "Plot out wit reference"
  model_info.Metrics.Description = ""
  model_info.Metrics.ComponentType = "metric"
  model_info.Experiments(1).Id = "1e1e735a-ca72-47f3-9e23-ef054322de06"
  model_info.Experiments(1).Name = "Five steps perturbed high noise"
  model_info.Experiments(1).Description = ""
  model_info.Experiments(1).ConstHorizonReference = 0
  model_info.Experiments(1).ComponentType = "scenario"
  model_info.Experiments(1).SimulationTime = 60
  model_info.Experiments(1).Subcomponents = "Disturbance"
  model_info.Experiments(1).Disturbance.Id = "d00b25fa-299c-4dde-a026-233da86bc131"
  model_info.Experiments(1).Disturbance.Name = ""
  model_info.Experiments(1).Disturbance.Description = ""
  model_info.Experiments(1).Disturbance.LibVersionHash = ""
  model_info.Experiments(1).Disturbance.Lib = "csbenchlab"
  model_info.Experiments(1).Disturbance.LibVersion = "0.0.1"
  model_info.Experiments(1).Disturbance.PluginType = "dist"
  model_info.Experiments(1).Disturbance.PluginName = "Gauss"
  model_info.Experiments(1).Disturbance.PluginImplementation = "mat"
  model_info.Experiments(1).Disturbance.ParentComponentId = "1e1e735a-ca72-47f3-9e23-ef054322de06"
  model_info.Experiments(1).Disturbance.ParentComponentName = "Five steps perturbed high noise"
  model_info.Experiments(1).Disturbance.ParentComponentType = "scenario"
  model_info.Experiments(1).Disturbance.ComponentType = "disturbance"
  model_info.Experiments(1).Disturbance.DestinationPath = "disturbances"
  model_info.Experiments(2).Id = "1e727098-795b-40af-9168-30502f01196e"
  model_info.Experiments(2).Name = "Two steps"
  model_info.Experiments(2).Description = ""
  model_info.Experiments(2).ConstHorizonReference = 0
  model_info.Experiments(2).ComponentType = "scenario"
  model_info.Experiments(2).SimulationTime = 60
  model_info.Experiments(2).Subcomponents = "Disturbance"
  model_info.Experiments(2).Disturbance = struct()
  model_info.Experiments(3).Id = "832a0fb6-0823-4b09-93b7-a1f8c841e784"
  model_info.Experiments(3).Name = "Sinuses"
  model_info.Experiments(3).Description = ""
  model_info.Experiments(3).ConstHorizonReference = 0
  model_info.Experiments(3).ComponentType = "scenario"
  model_info.Experiments(3).SimulationTime = 60
  model_info.Experiments(3).Subcomponents = "Disturbance"
  model_info.Experiments(3).Disturbance.Id = "6582568e-6a07-4ca1-973d-ce726013b9e5"
  model_info.Experiments(3).Disturbance.Name = ""
  model_info.Experiments(3).Disturbance.Description = ""
  model_info.Experiments(3).Disturbance.LibVersionHash = ""
  model_info.Experiments(3).Disturbance.Lib = "csbenchlab"
  model_info.Experiments(3).Disturbance.LibVersion = "0.0.1"
  model_info.Experiments(3).Disturbance.PluginType = "dist"
  model_info.Experiments(3).Disturbance.PluginName = "Gauss"
  model_info.Experiments(3).Disturbance.PluginImplementation = "mat"
  model_info.Experiments(3).Disturbance.ParentComponentId = "832a0fb6-0823-4b09-93b7-a1f8c841e784"
  model_info.Experiments(3).Disturbance.ParentComponentName = "Sinuses"
  model_info.Experiments(3).Disturbance.ParentComponentType = "scenario"
  model_info.Experiments(3).Disturbance.ComponentType = "disturbance"
  model_info.Experiments(3).Disturbance.DestinationPath = "disturbances"
  model_info.Experiments(4).Id = "85ae8ae8-3421-447e-86e6-f1860a57dbe5"
  model_info.Experiments(4).Name = "Two steps high noise"
  model_info.Experiments(4).Description = ""
  model_info.Experiments(4).ConstHorizonReference = 0
  model_info.Experiments(4).ComponentType = "scenario"
  model_info.Experiments(4).SimulationTime = 60
  model_info.Experiments(4).Subcomponents = "Disturbance"
  model_info.Experiments(4).Disturbance.Id = "ccaeaedb-34fb-4469-93e3-0e771cb356d7"
  model_info.Experiments(4).Disturbance.Name = "New Disturbance"
  model_info.Experiments(4).Disturbance.Description = ""
  model_info.Experiments(4).Disturbance.LibVersionHash = ""
  model_info.Experiments(4).Disturbance.Lib = "csbenchlab"
  model_info.Experiments(4).Disturbance.LibVersion = "0.0.1"
  model_info.Experiments(4).Disturbance.PluginType = "dist"
  model_info.Experiments(4).Disturbance.PluginName = "Gauss"
  model_info.Experiments(4).Disturbance.PluginImplementation = "mat"
  model_info.Experiments(4).Disturbance.ParentComponentId = "85ae8ae8-3421-447e-86e6-f1860a57dbe5"
  model_info.Experiments(4).Disturbance.ParentComponentType = "scenario"
  model_info.Experiments(4).Disturbance.ComponentType = "disturbance"
  model_info.Experiments(4).Disturbance.DestinationPath = "disturbances"
  model_info.Experiments(4).Disturbance.ParentComponentName = "Two steps high noise"
  model_info.Experiments(5).Id = "9caafca7-6b3d-4fd5-b43b-2d0badebda60"
  model_info.Experiments(5).Name = "Five steps perturbed"
  model_info.Experiments(5).Description = ""
  model_info.Experiments(5).ConstHorizonReference = 0
  model_info.Experiments(5).ComponentType = "scenario"
  model_info.Experiments(5).SimulationTime = 60
  model_info.Experiments(5).Subcomponents = "Disturbance"
  model_info.Experiments(5).Disturbance.Id = "941af73e-12e7-42cf-853d-f79bb40068e7"
  model_info.Experiments(5).Disturbance.Name = ""
  model_info.Experiments(5).Disturbance.Description = ""
  model_info.Experiments(5).Disturbance.LibVersionHash = ""
  model_info.Experiments(5).Disturbance.Lib = "csbenchlab"
  model_info.Experiments(5).Disturbance.LibVersion = "0.0.1"
  model_info.Experiments(5).Disturbance.PluginType = "dist"
  model_info.Experiments(5).Disturbance.PluginName = "Gauss"
  model_info.Experiments(5).Disturbance.PluginImplementation = "mat"
  model_info.Experiments(5).Disturbance.ParentComponentId = "9caafca7-6b3d-4fd5-b43b-2d0badebda60"
  model_info.Experiments(5).Disturbance.ParentComponentName = "Five steps perturbed"
  model_info.Experiments(5).Disturbance.ParentComponentType = "scenario"
  model_info.Experiments(5).Disturbance.ComponentType = "disturbance"
  model_info.Experiments(5).Disturbance.DestinationPath = "disturbances"
  model_info.Experiments(6).Id = "d997722b-b22e-4a88-a68f-d421073cfd81"
  model_info.Experiments(6).Name = "Sinuses high noise"
  model_info.Experiments(6).Description = ""
  model_info.Experiments(6).ConstHorizonReference = 0
  model_info.Experiments(6).ComponentType = "scenario"
  model_info.Experiments(6).SimulationTime = 60
  model_info.Experiments(6).Subcomponents = "Disturbance"
  model_info.Experiments(6).Disturbance.Id = "e3fab669-38a8-480e-9185-300544970487"
  model_info.Experiments(6).Disturbance.Name = ""
  model_info.Experiments(6).Disturbance.Description = ""
  model_info.Experiments(6).Disturbance.LibVersionHash = ""
  model_info.Experiments(6).Disturbance.Lib = "csbenchlab"
  model_info.Experiments(6).Disturbance.LibVersion = "0.0.1"
  model_info.Experiments(6).Disturbance.PluginType = "dist"
  model_info.Experiments(6).Disturbance.PluginName = "Gauss"
  model_info.Experiments(6).Disturbance.PluginImplementation = "mat"
  model_info.Experiments(6).Disturbance.ParentComponentId = "d997722b-b22e-4a88-a68f-d421073cfd81"
  model_info.Experiments(6).Disturbance.ParentComponentName = "Sinuses high noise"
  model_info.Experiments(6).Disturbance.ParentComponentType = "scenario"
  model_info.Experiments(6).Disturbance.ComponentType = "disturbance"
  model_info.Experiments(6).Disturbance.DestinationPath = "disturbances"
  model_info.Path = '/home/luka/fer/csbenchlab_gym/envs/marine_otter_full'
  model_info.IsControlEnvironment = 0
  model_type = 'scenario'
  old_params : object (value not decoded)
undefined symbols (not defined in the file): rpp_params
libraries: data_driven_lib_ctl x1, marine_lib_sys x1, cmmi_lib x1
PostSaveFcn:
  | on_model_save
settings Model: DataDictionary=RPP_BankedDeePC_bus_types.sldd  Creator=luka  LastModifiedBy=luka

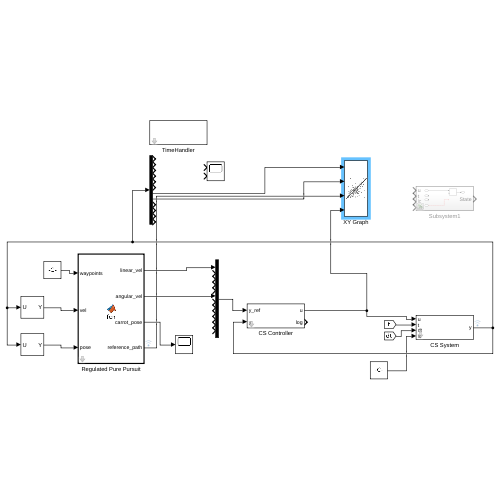
[thumbnail: Simulink's stored preview of the top-level diagram]
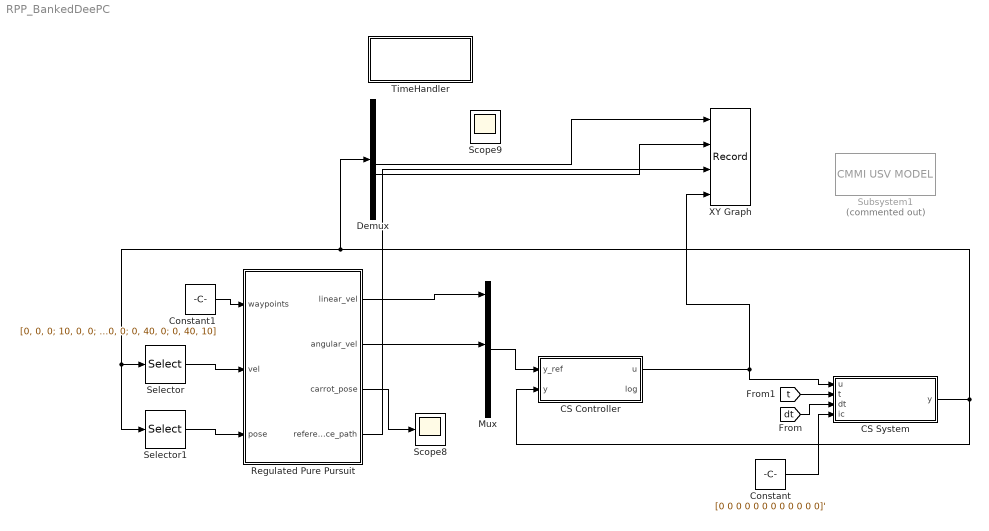
== system RPP_BankedDeePC ==
  CS Controller : Subsystem  Tag=__cs_template;__cs_comptype:ctl
      mask DialogControl ParameterGroupVar Prompt: Params
  CS System : Subsystem  Tag=__cs_template;__cs_comptype:sys
      mask DialogControl ParameterGroupVar Prompt: Params
  Constant : Constant  Value=[0 0 0 0 0 0 0 0 0 0 0 0]'
  Constant1 : Constant  Value=[0, 0, 0; 10, 0, 0; 10 10, 0; 0, 10, 0; 0, 20, 0; 10, 20, 0; 10, 30, 0; 0, 30, 0; 0, 40, 0; 0, 40, 10]
  Demux : Demux  Outputs=12
  Mux : Mux  Inputs=12
  Regulated Pure Pursuit : MATLAB Function  TreatAsAtomicUnit=on  mask{params=rpp_params}
  Scope8 : Scope
  Scope9 : Scope  NumInputPorts=2
  Selector : Selector  InputPortWidth=12  IndexOptions=Index vector (dialog)  Indices=[1 2 6]  OutputSizes=1
  Selector1 : Selector  InputPortWidth=12  IndexOptions=Index vector (dialog)  Indices=[7 8 12]  OutputSizes=1
  Subsystem1 : cmmi_lib/CMMI USV MODEL  Commented=on  SystemSampleTime=-1  VariantActivationTime=update diagram  AllowFlexibleInterface=on  Latency=0  AutoFrameSizeCalculation=off
      link override Subsystem/Saturation: UpperLimit=1  LowerLimit=-1
  TimeHandler : Subsystem
      mask DialogControl ParameterGroupVar Prompt: Params
  XY Graph : Record  FileSettingsInternal="{\"entries\":[{\"content\":{\"excelSettings\":{\"content\":{},\"type\":\"Streamout.ExcelSettings\"}},\"type\":\"Streamout.FileSettingStorage\",\"uuid\":\"\"}],\"packageUris\":[\"http:\\/\\/schema.mathworks.com\\/mf0\\/streamout_blocks\\/R2020a\"],\"version\":\"1.0\"}"  Layout=[1 1]  SignalsInternal="{\"entries\":[{\"content\":{\"signals\":[{\"content\":{\"blockPath\":[],\"dimensions\":[1],\"domain\":\"\",\"lineColor\":\"#a2142f\",\"lineWidth\":2,\"plots\":[ 1 ],\"port\":1,\"sid\":[\"\"],\"signalID\":1,\"signalName\":\"Demux:7\"},\"type\":\"RecordBlkView.Signal\",\"uuid\":\"\"},{\"content\":{\"blockPath\":[],\"dimensions\":[1],\"domain\":\"\",\"lineColor\":\"#139fff\",\"lineWidth\":2,\"plots\":[ 1 ],\"port\":2,\"sid\":[\"\"],\"signalID\":2,\"signalName\":\"Demux:8\"},\"type\":\"RecordBlkView.Signal\",\"uuid\":\"\"},{\"content\":{\"blockPath\":[],\"dimensions\":[901,3],\"domain\":\"\",\"hasChildren\":true,\"lineColor\":\"#ff6929\",\"lineWidth\":2,\"port\":3,\"sid\":[\"\"],\"signalID\":3,\"signalName\":\"Regulated Pure Pursuit:4\"},\"type\":\"RecordBlkView.Signal\",\"uuid\":\"\"},{\"content\":{\"blockPath\":[],\"channel\":[1,1],\"dimensions\":[901,3],\"domain\":\"\",\"lineColor\":\"#b746ff\",\"lineWidth\":2,\"parentID\":3,\"port\":3,\"sid\":[\"\"],\"signalID\":4,\"signalName\":\"Regulated Pure Pursuit:4\"},\"type\":\"RecordBlkView.Signal\",\"uuid\":\"\"},{\"content\":{\"blockPath\":[],\"dimensions\":[2],\"domain\":\"\",\"hasChildren\":true,\"lineColor\":\"#64d413\",\"lineWidth\":2,\"port\":4,\"sid\":[\"\"],\"signalID\":5,\"signalName\":\"CS Controller:1\"},\"type\":\"RecordBlkView.Signal\",\"uuid\":\"\"},{\"content\":{\"blockPath\":[],\"channel\":[1],\"dimensions\":[2],\"domain\":\"\",\"lineColor\":\"#ff13a6\",\"lineWidth\":2,\"parentID\":5,\"port\":4,\"sid\":[\"\"],\"signalID\":6,\"signalName\":\"CS Controller:1\"},\"type\":\"RecordBlkView.Signal\",\"uuid\":\"\"},{\"content\":{\"blockPath\":[],\"channel\":[2],\"dimensions\":[2],\"domain\":\"\",\"lineColor\":\"#77ac30\",\"lineWidth\":2,\"parentID\":5,\"port\":4,\"sid\":[\"\"],\"signalID\":7,\"signalName\":\"CS Controller:1\"},\"type\":\"RecordBlkView.Signal\",\"uuid\":\"\"}]},\"type\":\"RecordBlkView.InputSignals\",\"uuid\":\"\"}],\"packageUris\":[\"http:\\/\\/schema.mathworks.com\\/mf0\\/streamout_blocks\\/R2020a\"],\"version\":\"1.0\"}"  VisualizationBindings="{\"xyplotplugin\":{\"info\":[{\"series\":[{\"bindingParametersList\":[{\"parameter\":\"X-Axis\",\"signalID\":1,\"signalName\":\"Demux:7\"},{\"parameter\":\"Y-Axis\",\"signalID\":2,\"signalName\":\"Demux:8\"}],\"seriesID\":0}],\"subplotID\":1}]}}"  CompatibilityTag=XY
  wires:
  Constant1/1 -> Regulated Pure Pursuit/1(waypoints)
  Selector/1 -> Regulated Pure Pursuit/2(vel)
  Selector1/1 -> Regulated Pure Pursuit/3(pose)
  Regulated Pure Pursuit/3(carrot_pose) -> Scope8/1
  CS Controller/1(u) -> CS System/1(u), XY Graph/4
  [dt] -> CS System/3(dt)
  [t] -> CS System/2(t)
  Constant/1 -> CS System/4(ic)
  CS System/1(y) -> CS Controller/2(y), Selector1/1, Selector/1, Demux/1
  Regulated Pure Pursuit/4(reference_path) -> XY Graph/3
  Demux/7 -> XY Graph/1
  Demux/8 -> XY Graph/2
  Regulated Pure Pursuit/1(linear_vel) -> Mux/1
  Mux/1 -> CS Controller/1(y_ref)
  Regulated Pure Pursuit/2(angular_vel) -> Mux/6

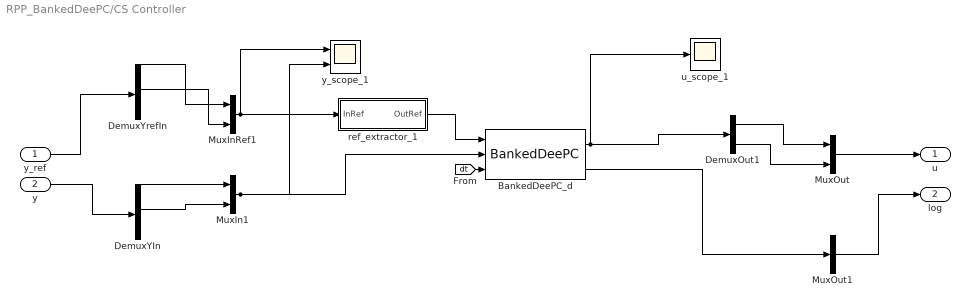
== system RPP_BankedDeePC/CS Controller ==
  y_ref : Inport  PortDimensions=12
  y : Inport  Port=2  PortDimensions=12
  BankedDeePC_d : data_driven_lib_ctl/BankedDeePC  Tag=__cs_comptype:ctl;__cs_compimpl:mat;  iid__=[57 99 52 48 98 97 52 48 45 97 51 48 99 45 52 100 52 55 45 98 54 101 97 45 51 51 50 100 53 51 48 56 53 100 98 52]  pid__=[66 97 110 107 101 100 68 101 101 80 67 58 100 97 116 97 95 100 114 105 118 101 110 95 108 105 98]  params=RPP_BankedDeePC_params.ctl.BankedDeePC_d  LogEntryType=RPP_BankedDeePC_CS_Controller_BankedDeePC_d_LT  data=RPP_BankedDeePC_CS_Controller_BankedDeePC_d_data  ParamsType=RPP_BankedDeePC_CS_Controller_BankedDeePC_d_PT  DataType=RPP_BankedDeePC_CS_Controller_BankedDeePC_d_DT  u_ic=[0;0]
  DemuxOut1 : Demux  Outputs=2
  DemuxYIn : Demux  Outputs=12
  DemuxYrefIn : Demux  Outputs=12
  MuxIn1 : Mux  Inputs=2
  MuxInRef1 : Mux  Inputs=2
  MuxOut : Mux  Inputs=2
  MuxOut1 : BusCreator  Inputs=1
  ref_extractor_1 : Subsystem
  u_scope_1 : Scope
  y_scope_1 : Scope  NumInputPorts=2
  u : Outport  PortDimensions=2
  log : Outport  Port=2
  wires:
  [dt] -> BankedDeePC_d/3
  y/1 -> DemuxYIn/1
  y_ref/1 -> DemuxYrefIn/1
  MuxOut/1 -> u/1
  MuxOut1/1 -> log/1
  MuxInRef1/1 -> ref_extractor_1/1(InRef), y_scope_1/1
  ref_extractor_1/1(OutRef) -> BankedDeePC_d/1
  MuxIn1/1 -> BankedDeePC_d/2, y_scope_1/2
  BankedDeePC_d/1 -> DemuxOut1/1, u_scope_1/1
  BankedDeePC_d/2 -> MuxOut1/1
  DemuxYIn/1 -> MuxIn1/1
  DemuxYrefIn/1 -> MuxInRef1/1
  DemuxYIn/6 -> MuxIn1/2
  DemuxYrefIn/6 -> MuxInRef1/2
  DemuxOut1/1 -> MuxOut/1
  DemuxOut1/2 -> MuxOut/2

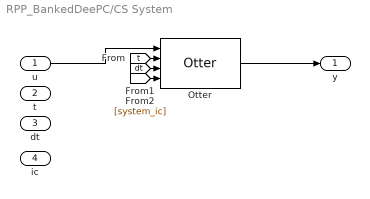
== system RPP_BankedDeePC/CS System ==
  u : Inport
  t : Inport  Port=2
  dt : Inport  Port=3
  ic : Inport  Port=4
  Otter : marine_lib_sys/Otter  Tag=system;__cs_slx_sys;__cs_comptype:sys;__cs_compimpl:slx;  payload_mass=RPP_BankedDeePC_params.sys.Otter.payload_mass  payload_location=RPP_BankedDeePC_params.sys.Otter.payload_location  current_speed=RPP_BankedDeePC_params.sys.Otter.current_speed  current_direction=RPP_BankedDeePC_params.sys.Otter.current_direction  out_gain=RPP_BankedDeePC_params.sys.Otter.out_gain  iid__=[52 97 48 100 49 48 49 48 45 52 53 52 57 45 52 100 53 49 45 98 51 97 53 45 54 48 50 101 55 99 57 51 50 98 52 53]  pid__=[79 116 116 101 114 58 109 97 114 105 110 101 95 108 105 98]  params=ActiveExperiment.SystemParams  params_struct_name=RPP_BankedDeePC_params.sys.Otter
  y : Outport
  wires:
  u/1 -> Otter/1
  Otter/1 -> y/1
  [t] -> Otter/2
  [dt] -> Otter/3
  [system_ic] -> Otter/4

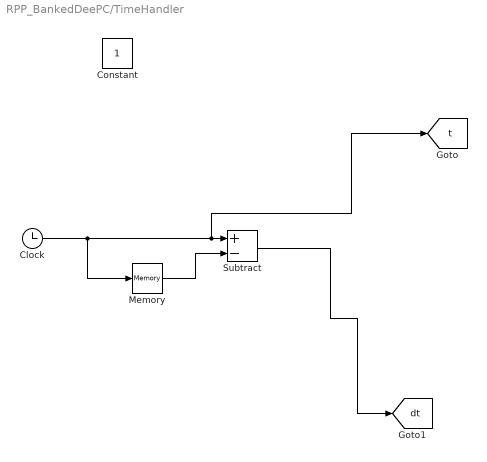
== system RPP_BankedDeePC/TimeHandler ==
  Clock : Clock
  Constant : Constant
  Memory : Memory
  Subtract : Sum  Inputs=+-
  tag scope: dt=global, t=global
  wires:
  Clock/1 -> [t], Subtract/1, Memory/1
  Memory/1 -> Subtract/2
  Subtract/1 -> [dt]

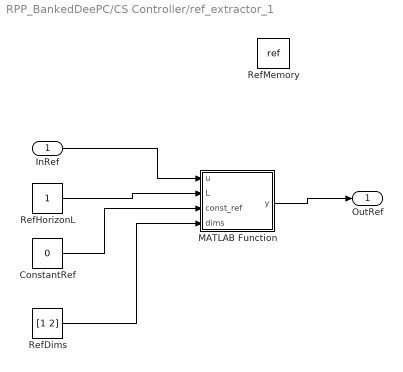
== system RPP_BankedDeePC/CS Controller/ref_extractor_1 ==
  InRef : Inport
  ConstantRef : Constant  Value=0
  MATLAB Function : MATLAB Function  TreatAsAtomicUnit=on
  RefDims : Constant  Value=[1 2]
  RefHorizonL : Constant
  RefMemory : DataStoreMemory  DataStoreName=ref  WriteAfterWriteMsg=warning  ShowAdditionalParam=off  OutDataTypeStr=double
  OutRef : Outport
  wires:
  ConstantRef/1 -> MATLAB Function/3(const_ref)
  RefDims/1 -> MATLAB Function/4(dims)
  RefHorizonL/1 -> MATLAB Function/2(L)
  InRef/1 -> MATLAB Function/1(u)
  MATLAB Function/1(y) -> OutRef/1

== matlab function RPP_BankedDeePC/Regulated Pure Pursuit ==
  settings: updateMethod=DISCRETE
  data: waypoints input; vel input; pose input; linear_vel output; params parameter; angular_vel output; carrot_pose output size=[1 3]; reference_path output
function [linear_vel, angular_vel, carrot_pose, reference_path] = fcn(waypoints, vel, pose, params)

    persistent global_path idx initial_global_path
    use_waypoints = 0;
    num_divs = 100;        
    if isempty(global_path)

        if use_waypoints
            global_path = zeros((height(waypoints)-1) * num_divs+1, 3);
            global_path(1, :) = waypoints(1, :);
            for i=1:length(waypoints)-1
                global_path(2 + (i-1)*num_divs : i*num_divs+1, :) = get_traj_between(waypoints(i, :), waypoints(i+1, :), num_divs);
            end
            idx = 1;
        else
            global_path = zeros((height(waypoints)-1) * num_divs+1, 3);
            global_path(1, :) = waypoints(1, :);
            k=5;
            kx=1.3;
            ky=0;
            L = 200;
            N = 5;
            theta=linspace(0, 2*N*pi, L);
            r = k*theta;
            x = k*(cos(theta)-1) + kx*theta;
            y = k*sin(theta) + ky*theta;
            global_path(2:L+1, :) = [x' y' zeros(L, 1)] + repmat(global_path(1, :), L, 1);
            global_path(L+2:end, :) = repmat(global_path(L+1, :), length(global_path) - L-1, 1);
            idx = 1;
        end
        initial_global_path = global_path;
    end
    reference_path = initial_global_path;
    coder.extrinsic('regulated_pure_pursuit')
    coder.extrinsic('transform_path_to_local')
    coder.extrinsic('prune_global_path')
    linear_vel = 0; angular_vel = 0;
    carrot_pose = [0,0,0];
    idx = prune_global_path(pose, global_path, idx, 0.8 * params.lookahead_dist, 2);
    local_path = transform_path_to_local(pose, global_path(idx:end, :));
    [linear_vel, angular_vel, carrot] = regulated_pure_pursuit(local_path, vel, params);
    carrot_pose(1:2) = carrot;
end

== matlab function RPP_BankedDeePC/CS Controller/ref_extractor_1/MATLAB Function ==
  settings: updateMethod=DISCRETE
  data: u input; L input; const_ref input; dims input; y output; ref data_store_memory; GlobalReference parameter
function y = fcn(u, L, const_ref, dims, GlobalReference)

persistent cnt
global ref

if isempty(cnt)
    cnt = 0;
end

if GlobalReference == 0
    y = repmat(u', 1);
    return;
end


cnt = cnt+1;

horizon_end = cnt+L-1;
if L > 1 
   if horizon_end > length(GlobalReference)
        if size(ref, 1) == size(u, 1)
            y = permute(ref, [2, 1]);
        else
            y = ref;
        end       
        return
   end

   if size(ref, 1) == size(u, 1)
      
      if const_ref == 0
        ref(:, :) = GlobalReference(cnt:horizon_end, dims)';
      else
        ref(:, :) = repmat(GlobalReference(cnt, dims)', 1, L);
      end
      y = permute(ref, [2, 1]);
   else
      if const_ref == 0
        ref(1:L, :) = GlobalReference(cnt:horizon_end, dims);
      else
        ref(1:L, :) = repmat(GlobalReference(cnt, dims), L, 1);
      end
      y = ref;
   end
else
   if size(ref, 1) == size(u, 1)
       ref = u;
       y = permute(ref, [2, 1]);
   else
      ref(1, :) = u';
      y = ref;
   end
end
